simulink model "oil_withC2"  (R2023b)
settings: Solver=VariableStepAuto  StartTime=0.0  StopTime=1.04  RelTol=1e-3
undefined symbols (not defined in the file or in its folder): kc, tc
settings Model: Creator=olavhegg  LastModifiedBy=olavhegg

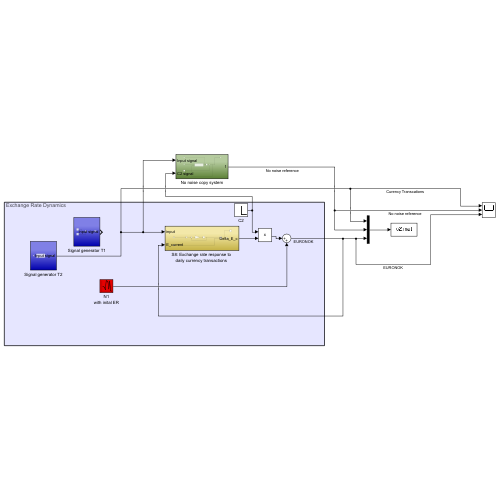
[thumbnail: Simulink's stored preview of the top-level diagram]
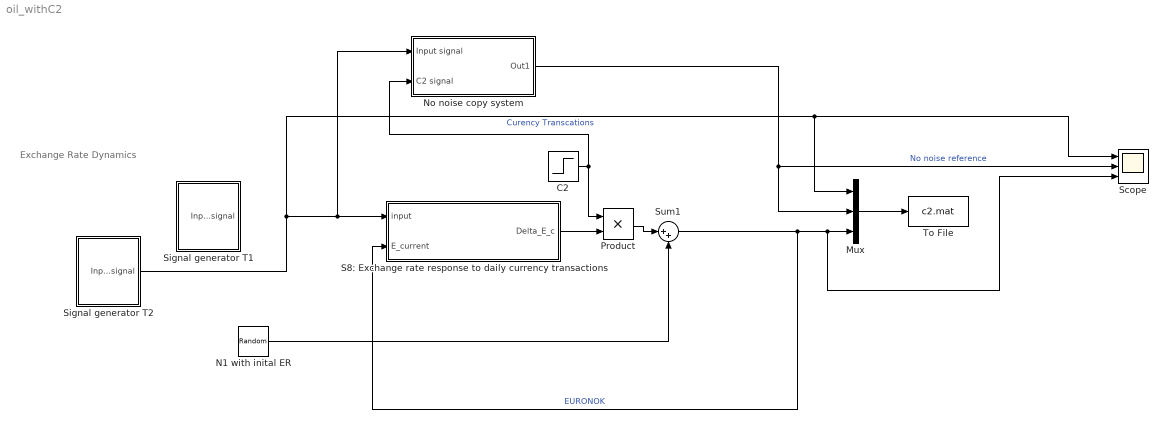
== system oil_withC2 ==
  note: Exchange Rate Dynamics
  C2 : Step  Time=0.38  Before=1  After=0  SampleTime=0
  Mux : Mux  Inputs=3
  N1 with inital ER : RandomNumber  Mean=12  Variance=0.00001259  Seed=23341  SampleTime=0.00142857
  No noise copy system : Subsystem
  Product : Product
  "S8: Exchange rate response to daily currency transactions " : Subsystem
  Scope : Scope  NumInputPorts=3
  Signal generator T1 : Subsystem
  Signal generator T2 : Subsystem
  Sum1 : Sum  Inputs=|++
  To File : ToFile  Filename=c2.mat  MatrixName=c2  SampleTime=0.0001
  wires:
  Product/1 -> Sum1/1
  N1 with inital ER/1 -> Sum1/2
  Sum1/1 -> "S8: Exchange rate response to daily currency transactions "/2(E_current), Scope/3, Mux/3  "EURONOK"
  No noise copy system/1(Out1) -> Scope/2, Mux/2  "No noise reference"
  Mux/1 -> To File/1
  Signal generator T2/1(Input signal) -> Mux/1, Scope/1, "S8: Exchange rate response to daily currency transactions "/1(input), No noise copy system/1(Input signal)  "Curency Transcations"
  "S8: Exchange rate response to daily currency transactions "/1(Delta_E_c) -> Product/2
  C2/1 -> Product/1, No noise copy system/2(C2 signal)

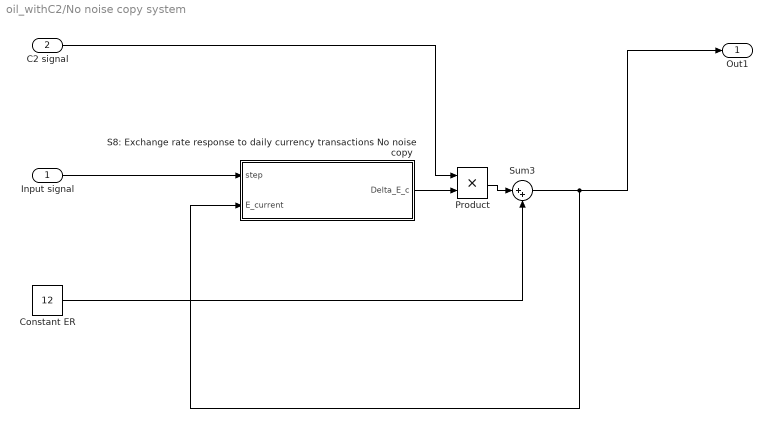
== system oil_withC2/No noise copy system ==
  Input signal : Inport
  C2 signal : Inport  Port=2
  Constant ER : Constant  Value=12
  Product : Product
  S8: Exchange rate response to daily currency transactions No noise copy : Subsystem
  Sum3 : Sum  Inputs=|++
  Out1 : Outport
  wires:
  Constant ER/1 -> Sum3/2
  S8: Exchange rate response to daily currency transactions No noise copy/1(Delta_E_c) -> Product/2
  Sum3/1 -> S8: Exchange rate response to daily currency transactions No noise copy/2(E_current), Out1/1
  Input signal/1 -> S8: Exchange rate response to daily currency transactions No noise copy/1(step)
  Product/1 -> Sum3/1
  C2 signal/1 -> Product/1

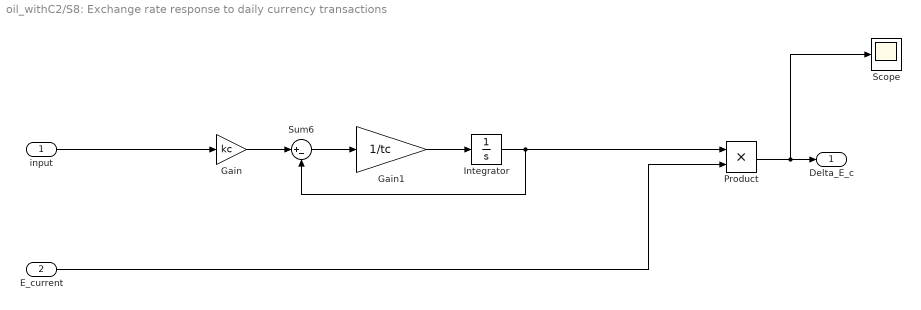
== system oil_withC2/S8: Exchange rate response to daily currency transactions  ==
  input : Inport
  E_current : Inport  Port=2
  Gain : Gain  Gain=kc
  Gain1 : Gain  Gain=1/tc
  Integrator : Integrator
  Product : Product
  Scope : Scope
  Sum6 : Sum  Inputs=|+-
  Delta_E_c : Outport
  wires:
  Gain/1 -> Sum6/1
  Gain1/1 -> Integrator/1
  Sum6/1 -> Gain1/1
  input/1 -> Gain/1
  Integrator/1 -> Product/1, Sum6/2
  E_current/1 -> Product/2
  Product/1 -> Scope/1, Delta_E_c/1

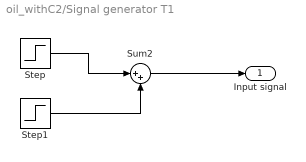
== system oil_withC2/Signal generator T1 ==
  Step : Step  Time=0.1  After=500  SampleTime=0
  Step1 : Step  Time=0.11  After=-500  SampleTime=0
  Sum2 : Sum  Inputs=|++
  Input signal : Outport
  wires:
  Sum2/1 -> Input signal/1
  Step1/1 -> Sum2/2
  Step/1 -> Sum2/1

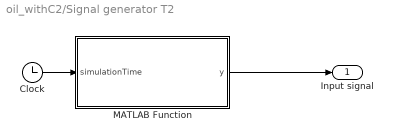
== system oil_withC2/Signal generator T2 ==
  Clock : Clock
  MATLAB Function : MATLAB Function  TreatAsAtomicUnit=on  SystemSampleTime=0.0001
  Input signal : Outport
  wires:
  Clock/1 -> MATLAB Function/1(simulationTime)
  MATLAB Function/1(y) -> Input signal/1

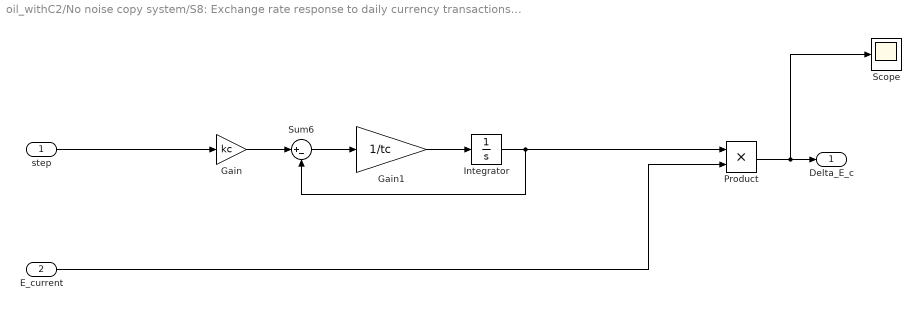
== system oil_withC2/No noise copy system/S8: Exchange rate response to daily currency transactions No noise copy ==
  step : Inport
  E_current : Inport  Port=2
  Gain : Gain  Gain=kc
  Gain1 : Gain  Gain=1/tc
  Integrator : Integrator
  Product : Product
  Scope : Scope
  Sum6 : Sum  Inputs=|+-
  Delta_E_c : Outport
  wires:
  Gain/1 -> Sum6/1
  Gain1/1 -> Integrator/1
  Sum6/1 -> Gain1/1
  step/1 -> Gain/1
  Integrator/1 -> Product/1, Sum6/2
  E_current/1 -> Product/2
  Product/1 -> Scope/1, Delta_E_c/1

== matlab function oil_withC2/Signal generator T2/MATLAB Function ==
  data: y output; simulationTime input
function y = historicTransactions(simulationTime)

persistent values;
persistent currentIndex;
persistent lastSimulationTime;

% Define the values if not already defined
if isempty(values)
    values = [-250, 0, 0, 2000, 2000, 1500, 1500, 1500, 3500, 4300, 3700, 1900];
end

% Initialize currentIndex if not already initialized
if isempty(currentIndex)
    currentIndex = 1;
end

% Initialize lastSimulationTime if not already initialized
if isempty(lastSimulationTime)
    lastSimulationTime = 0;
end

% Determine the index based on simulation time and timestep
timestep = 0.52/12; % Timestep in seconds
if simulationTime >= lastSimulationTime + timestep
    currentIndex = mod(floor(simulationTime / timestep), length(values)) + 1;
    lastSimulationTime = floor(simulationTime / timestep) * timestep;
end

% Output current value
y = values(currentIndex);

end
